simulink model "Plant"  (R2021a)
settings: Solver=VariableStepAuto  StartTime=0.0  StopTime=10.0  RelTol=1e-3
values from neighbouring files (symbols this model uses):
  Jm = M*g*L/vm0/(Km/taum)    (= 0.00129122601065)    [Clay_Plant_Setup.m]
  Jp = L^2*M    (= 0.0021040464375)    [Clay_Plant_Setup.m]
  KcRa = M*g*L/vm0    (= 0.109014347826)    [Clay_Plant_Setup.m]
  Km = 23.133    [Clay_Plant_Setup.m]
undefined symbols (not defined in the file or in its folder): g_n, Ka_fit, Kp_tuned, Kt, L_n, M_n, N_n, x0
libraries: simulink x1, simulink_extras x1
settings Model: Creator=domin  LastModifiedBy=domin
settings ModelReferenceCC: ModelReferenceNumInstancesAllowed=Single

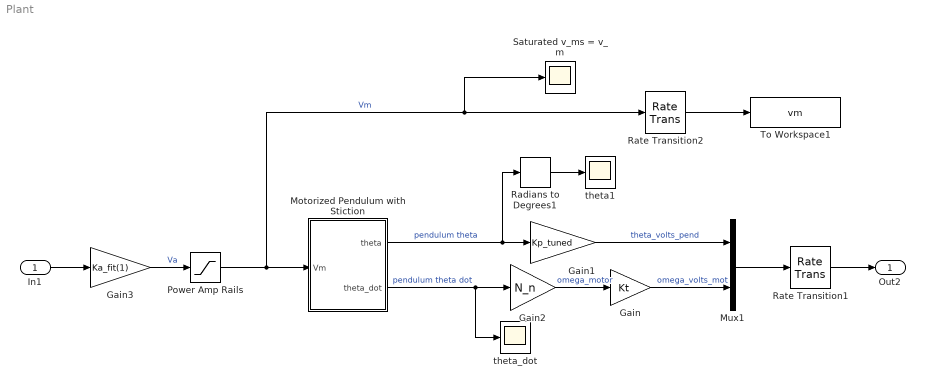
== system Plant ==
  In1 : Inport  SampleTime=.01
  Gain : Gain  Gain=Kt
  Gain1 : Gain  Gain=Kp_tuned
  Gain2 : Gain  Gain=N_n
  Gain3 : Gain  Gain=Ka_fit(1)
  Motorized Pendulum with Stiction : Subsystem
  Mux1 : Mux  Inputs=2
  Power Amp Rails : Saturate  UpperLimit=15  LowerLimit=-15
  Radians to Degrees1 : simulink_extras/Transformations/Radians to Degrees
  Rate Transition1 : RateTransition  InitialCondition=x0  OutPortSampleTime=0.01
  Rate Transition2 : RateTransition  OutPortSampleTime=0
  Saturated v_ms = v_m : Scope
  To Workspace1 : ToWorkspace  VariableName=vm  SampleTime=-1
  theta1 : Scope
  theta_dot : Scope
  Out2 : Outport
  wires:
  Power Amp Rails/1 -> Rate Transition2/1, Saturated v_ms = v_m/1, Motorized Pendulum with Stiction/1(Vm)  "Vm"
  In1/1 -> Gain3/1
  Gain3/1 -> Power Amp Rails/1  "Va"
  Gain1/1 -> Mux1/1  "theta_volts_pend"
  Gain/1 -> Mux1/2  "omega_volts_mot"
  Gain2/1 -> Gain/1  "omega_motor"
  Motorized Pendulum with Stiction/2(theta_dot) -> theta_dot/1, Gain2/1  "pendulum theta dot"
  Motorized Pendulum with Stiction/1(theta) -> Radians to Degrees1/1, Gain1/1  "pendulum theta"
  Radians to Degrees1/1 -> theta1/1
  Rate Transition1/1 -> Out2/1
  Mux1/1 -> Rate Transition1/1
  Rate Transition2/1 -> To Workspace1/1

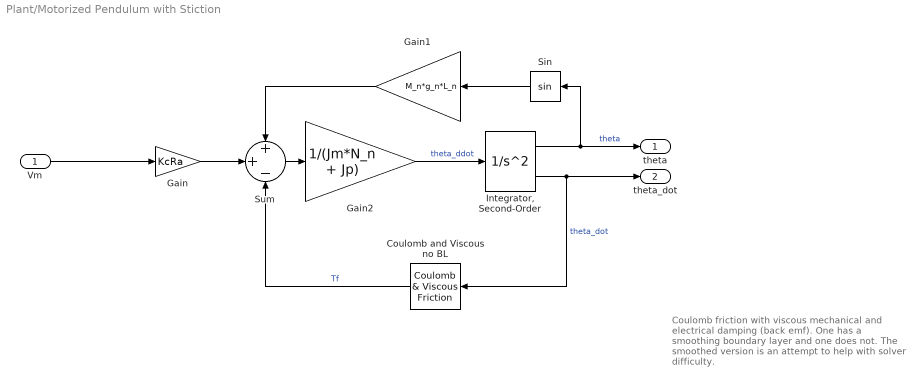
== system Plant/Motorized Pendulum with Stiction ==
  note: Coulomb friction with viscous mechanical
      | and electrical damping (back emf). One has a
      | smoothing boundary layer and one does not.
      | The smoothed version is an attempt to help with
      | solver difficulty.
  Vm : Inport
  Coulomb and Viscous no BL : simulink/Discontinuities/Coulomb & Viscous Friction  offset=T_ba_n  gain=N_n*KcRa/Km
  Gain : Gain  Gain=KcRa
  Gain1 : Gain  Gain=M_n*g_n*L_n
  Gain2 : Gain  Gain=1/(Jm*N_n + Jp)
  "Integrator, Second-Order" : SecondOrderIntegrator  ICX=x0(1)  ICDXDT=x0(2)  ZeroCross=off
  Sin : Trigonometry
  Sum : Sum  Inputs=++-
  theta : Outport
  theta_dot : Outport  Port=2
  wires:
  Gain2/1 -> "Integrator, Second-Order"/1  "theta_ddot"
  Sin/1 -> Gain1/1
  "Integrator, Second-Order"/2 -> theta_dot/1, Coulomb and Viscous no BL/1  "theta_dot"
  "Integrator, Second-Order"/1 -> Sin/1, theta/1  "theta"
  Gain1/1 -> Sum/1
  Sum/1 -> Gain2/1
  Vm/1 -> Gain/1
  Gain/1 -> Sum/2
  Coulomb and Viscous no BL/1 -> Sum/3  "Tf"
